simulink model "sim_p_regler_ideale_strecke"  (R2016b)
settings: Solver=FixedStepAuto  StartTime=0.0  StopTime=20  FixedStep=0.001  RelTol=1e-3
undefined symbols (not defined in the file or in its folder): transfunc
settings Model: Creator=Fritz  LastModifiedBy=Fritz

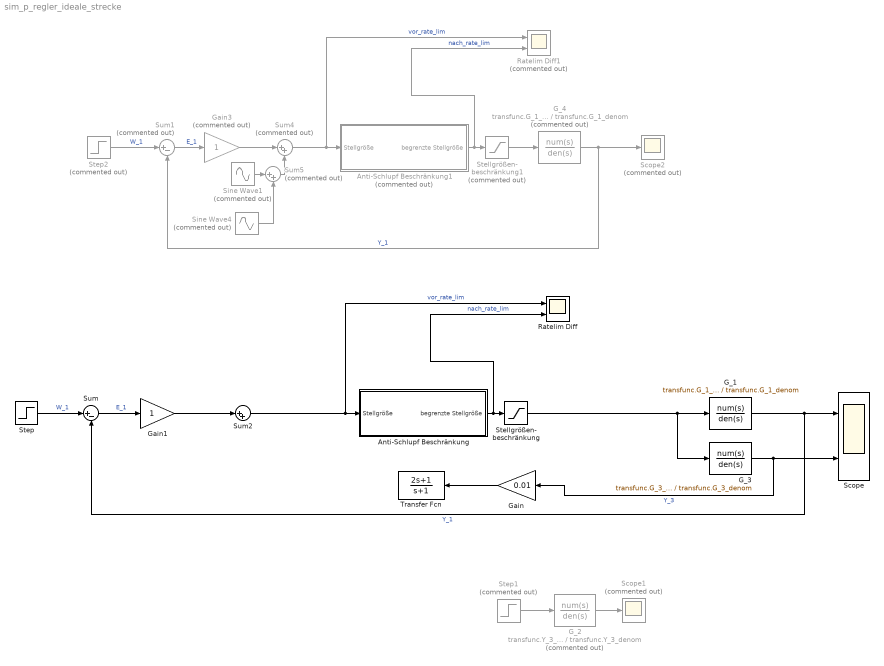
== system sim_p_regler_ideale_strecke ==
  Anti-Schlupf Beschränkung : Subsystem
  Anti-Schlupf Beschränkung1 : Subsystem  Commented=on
  G_1 : TransferFcn  Numerator=transfunc.G_1_numer  Denominator=transfunc.G_1_denom
  G_2 : TransferFcn  Commented=on  Numerator=transfunc.Y_3_numer  Denominator=transfunc.Y_3_denom
  G_3 : TransferFcn  Numerator=transfunc.G_3_numer  Denominator=transfunc.G_3_denom
  G_4 : TransferFcn  Commented=on  Numerator=transfunc.G_1_numer  Denominator=transfunc.G_1_denom
  Gain : Gain  Gain=0.01
  Gain1 : Gain
  Gain3 : Gain  Commented=on
  Ratelim Diff : Scope  NumInputPorts=2
  Ratelim Diff1 : Scope  Commented=on  NumInputPorts=2
  Scope : Scope  NumInputPorts=2
  Scope1 : Scope  Commented=on
  Scope2 : Scope  Commented=on
  Sine Wave1 : Sin  Commented=on  Amplitude=0.2  Frequency=4.43  SampleTime=0
  Sine Wave4 : Sin  Commented=on  Amplitude=0.2  Frequency=9.9  SampleTime=0
  Stellgrößen- beschränkung : Saturate  UpperLimit=1  LowerLimit=-1
  Stellgrößen- beschränkung1 : Saturate  Commented=on  UpperLimit=1  LowerLimit=-1
  Step : Step  Time=0  SampleTime=0
  Step1 : Step  Commented=on  SampleTime=0
  Step2 : Step  Commented=on  Time=0  SampleTime=0
  Sum : Sum  Inputs=|+-
  Sum1 : Sum  Commented=on  Inputs=|+-
  Sum2 : Sum  Inputs=|++
  Sum4 : Sum  Commented=on  Inputs=|++
  Sum5 : Sum  Commented=on  Inputs=|++
  Transfer Fcn : TransferFcn  Numerator=[2 1]  Denominator=[1 1]
  wires:
  G_3/1 -> Gain/1, Scope/2  "Y_3"
  Gain1/1 -> Sum2/1
  Sum/1 -> Gain1/1  "E_1"
  G_1/1 -> Scope/1, Sum/2  "Y_1"
  Step/1 -> Sum/1  "W_1"
  Anti-Schlupf Beschränkung/1(begrenzte Stellgröße) -> Ratelim Diff/2, Stellgrößen- beschränkung/1  "nach_rate_lim"
  Sum2/1 -> Ratelim Diff/1, Anti-Schlupf Beschränkung/1(Stellgröße)  "vor_rate_lim"
  Gain/1 -> Transfer Fcn/1
  G_2/1 -> Scope1/1
  Step1/1 -> G_2/1
  Stellgrößen- beschränkung/1 -> G_3/1, G_1/1
  Sum1/1 -> Gain3/1  "E_1"
  G_4/1 -> Scope2/1, Sum1/2  "Y_1"
  Step2/1 -> Sum1/1  "W_1"
  Anti-Schlupf Beschränkung1/1(begrenzte Stellgröße) -> Ratelim Diff1/2, Stellgrößen- beschränkung1/1  "nach_rate_lim"
  Sum4/1 -> Ratelim Diff1/1, Anti-Schlupf Beschränkung1/1(Stellgröße)  "vor_rate_lim"
  Stellgrößen- beschränkung1/1 -> G_4/1
  Gain3/1 -> Sum4/1
  Sine Wave1/1 -> Sum5/1
  Sine Wave4/1 -> Sum5/2
  Sum5/1 -> Sum4/2

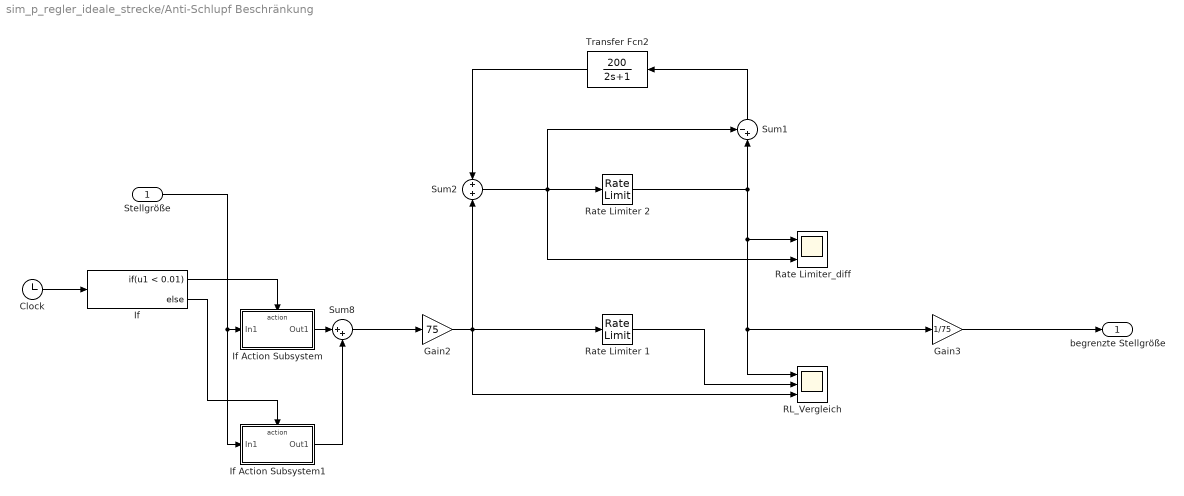
== system sim_p_regler_ideale_strecke/Anti-Schlupf Beschränkung ==
  Stellgröße : Inport
  Clock : Clock
  Gain2 : Gain  Gain=75
  Gain3 : Gain  Gain=1/75
  If : If  IfExpression=u1 < 0.01
  If Action Subsystem : Subsystem  TreatAsAtomicUnit=on
  If Action Subsystem1 : Subsystem  TreatAsAtomicUnit=on
  RL_Vergleich : Scope  NumInputPorts=3
  Rate Limiter 1 : RateLimiter  RisingSlewLimit=9.57  FallingSlewLimit=-9.57  SampleTimeMode=inherited
  Rate Limiter 2 : RateLimiter  RisingSlewLimit=9.57  FallingSlewLimit=-9.57  SampleTimeMode=inherited
  Rate Limiter_diff : Scope  NumInputPorts=2
  Sum1 : Sum  Inputs=-+|
  Sum2 : Sum  Inputs=+|+
  Sum8 : Sum  Inputs=|++
  Transfer Fcn2 : TransferFcn  Numerator=[200]  Denominator=[2 1]
  begrenzte Stellgröße : Outport
  wires:
  Stellgröße/1 -> If Action Subsystem1/1(In1), If Action Subsystem/1(In1)
  If Action Subsystem/1(Out1) -> Sum8/1
  If Action Subsystem1/1(Out1) -> Sum8/2
  Clock/1 -> If/1
  If/1 -> If Action Subsystem/Action
  If/2 -> If Action Subsystem1/Action
  Sum8/1 -> Gain2/1
  Sum2/1 -> Rate Limiter_diff/2, Sum1/1, Rate Limiter 2/1
  Sum1/1 -> Transfer Fcn2/1
  Transfer Fcn2/1 -> Sum2/1
  Rate Limiter 2/1 -> Gain3/1, RL_Vergleich/1, Rate Limiter_diff/1, Sum1/2
  Rate Limiter 1/1 -> RL_Vergleich/2
  Gain2/1 -> RL_Vergleich/3, Sum2/2, Rate Limiter 1/1
  Gain3/1 -> begrenzte Stellgröße/1

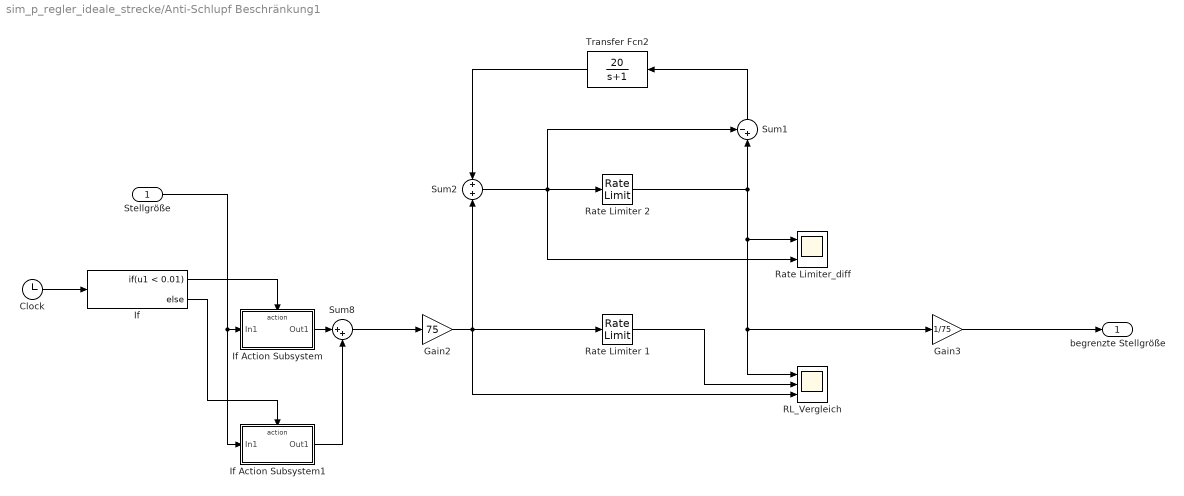
== system sim_p_regler_ideale_strecke/Anti-Schlupf Beschränkung1 ==
  Stellgröße : Inport
  Clock : Clock
  Gain2 : Gain  Gain=75
  Gain3 : Gain  Gain=1/75
  If : If  IfExpression=u1 < 0.01
  If Action Subsystem : Subsystem  TreatAsAtomicUnit=on
  If Action Subsystem1 : Subsystem  TreatAsAtomicUnit=on
  RL_Vergleich : Scope  NumInputPorts=3
  Rate Limiter 1 : RateLimiter  RisingSlewLimit=9.57  FallingSlewLimit=-9.57  SampleTimeMode=inherited
  Rate Limiter 2 : RateLimiter  RisingSlewLimit=9.57  FallingSlewLimit=-9.57  SampleTimeMode=inherited
  Rate Limiter_diff : Scope  NumInputPorts=2
  Sum1 : Sum  Inputs=-+|
  Sum2 : Sum  Inputs=+|+
  Sum8 : Sum  Inputs=|++
  Transfer Fcn2 : TransferFcn  Numerator=[20]  Denominator=[1 1]
  begrenzte Stellgröße : Outport
  wires:
  Stellgröße/1 -> If Action Subsystem1/1(In1), If Action Subsystem/1(In1)
  If Action Subsystem/1(Out1) -> Sum8/1
  If Action Subsystem1/1(Out1) -> Sum8/2
  Clock/1 -> If/1
  If/1 -> If Action Subsystem/Action
  If/2 -> If Action Subsystem1/Action
  Sum8/1 -> Gain2/1
  Sum2/1 -> Rate Limiter_diff/2, Sum1/1, Rate Limiter 2/1
  Sum1/1 -> Transfer Fcn2/1
  Transfer Fcn2/1 -> Sum2/1
  Rate Limiter 2/1 -> Gain3/1, RL_Vergleich/1, Rate Limiter_diff/1, Sum1/2
  Rate Limiter 1/1 -> RL_Vergleich/2
  Gain2/1 -> RL_Vergleich/3, Sum2/2, Rate Limiter 1/1
  Gain3/1 -> begrenzte Stellgröße/1

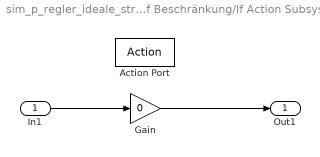
== system sim_p_regler_ideale_strecke/Anti-Schlupf Beschränkung/If Action Subsystem ==
  In1 : Inport
  Action Port : ActionPort  ActionType=then
  Gain : Gain  Gain=0
  Out1 : Outport
  wires:
  In1/1 -> Gain/1
  Gain/1 -> Out1/1

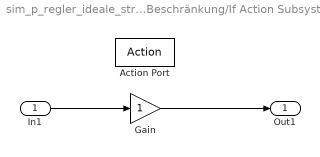
== system sim_p_regler_ideale_strecke/Anti-Schlupf Beschränkung/If Action Subsystem1 ==
  In1 : Inport
  Action Port : ActionPort  ActionType=else
  Gain : Gain
  Out1 : Outport
  wires:
  In1/1 -> Gain/1
  Gain/1 -> Out1/1

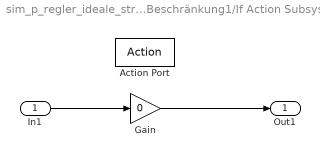
== system sim_p_regler_ideale_strecke/Anti-Schlupf Beschränkung1/If Action Subsystem ==
  In1 : Inport
  Action Port : ActionPort  ActionType=then
  Gain : Gain  Gain=0
  Out1 : Outport
  wires:
  In1/1 -> Gain/1
  Gain/1 -> Out1/1

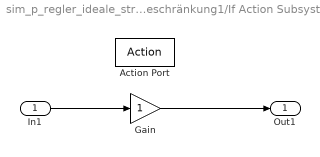
== system sim_p_regler_ideale_strecke/Anti-Schlupf Beschränkung1/If Action Subsystem1 ==
  In1 : Inport
  Action Port : ActionPort  ActionType=else
  Gain : Gain
  Out1 : Outport
  wires:
  In1/1 -> Gain/1
  Gain/1 -> Out1/1
